simulink model "SMC2"  (R2018b)
settings: Solver=VariableStepAuto  StartTime=0.0  StopTime=50  MaxStep=0.001  RelTol=1e-3  EnableMultiTasking=on
settings Model: Creator=omid_zandi  LastModifiedBy=Arash
settings OptimizationCC: LifeSpan=inf
settings DebuggingCC: SFUnexpectedBacktrackingDiag=warning  SFNoUnconditionalDefaultTransitionDiag=warning
settings SFSimCC: SimUseLocalCustomCode=off
settings RTWCC: RTWUseLocalCustomCode=off
settings CodeAppCC: StateflowObjectComments=on
settings GRTTargetCC: TargetLangStandard=C89/C90 (ANSI)  GeneratePreprocessorConditionals=Disable all
settings ConfigComp: CovMetricSettings=dw  CovHtmlReporting=on  CovSaveCumulativeToWorkspaceVar=on  CovSaveSingleToWorkspaceVar=on  CovExternalEMLEnable=off

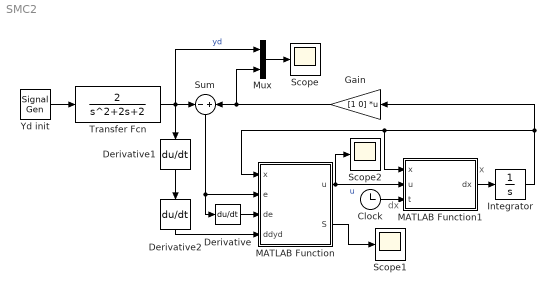
== system SMC2 ==
  note: dx
  note: x
  Clock : Clock
  Derivative : Derivative
  Derivative1 : Derivative
  Derivative2 : Derivative
  Gain : Gain  Gain=[1 0]  Multiplication=Matrix(K*u)
  Integrator : Integrator  InitialCondition=randn(2,1)
  MATLAB Function : MATLAB Function  TreatAsAtomicUnit=on
  MATLAB Function1 : MATLAB Function  TreatAsAtomicUnit=on
  Mux : Mux  Inputs=2
  Scope : Scope
  Scope1 : Scope
  Scope2 : Scope
  Sum : Sum  Inputs=-|+
  Transfer Fcn : TransferFcn  Numerator=[2]  Denominator="[1  2 2]"
  "Yd init " : SignalGenerator  WaveForm=square  Frequency=0.05
  wires:
  Integrator/1 -> MATLAB Function1/1(x), MATLAB Function/1(x), Gain/1
  MATLAB Function1/1(dx) -> Integrator/1
  MATLAB Function/1(u) -> Scope2/1, MATLAB Function1/2(u)  "u"
  Clock/1 -> MATLAB Function1/3(t)
  "Yd init "/1 -> Transfer Fcn/1
  Transfer Fcn/1 -> Mux/1, Derivative1/1, Sum/1  "yd"
  Gain/1 -> Mux/2, Sum/2
  Sum/1 -> MATLAB Function/2(e), Derivative/1
  Derivative/1 -> MATLAB Function/3(de)
  Derivative1/1 -> Derivative2/1
  Derivative2/1 -> MATLAB Function/4(ddyd)
  MATLAB Function/2(S) -> Scope1/1
  Mux/1 -> Scope/1

== matlab function SMC2/MATLAB Function1 ==
  data: x input; dx output; u input; t input
function dx = fcn(x , u , t)
%#codegen
dx = zeros(2,1) ;
dx(1) = x(2) ; 
dx(2) = x(1) * exp(-x(2)^2) + (1.5 + sin(t))*u ;

== matlab function SMC2/MATLAB Function ==
  data: x input; u output; S output; e input; de input; ddyd input
function [u , S] = fcn(x, e, de, ddyd)
k = 4;
eta = 4;
EPS = 0.01;
S = de  + k * e;
F = (abs(x(1)) + k * abs(x(2)) + abs(ddyd))/0.5;
% u = -(F + eta) * sign(S);
% u = -(F + eta) * S/(abs(S)  + EPS);
u = -(F + eta) * SAT(S);
end

% To avoid chattering
function  Z = SAT(S)
delta = 0.1;
if S > delta
    Z = 1;
elseif S < -delta
    Z = -1;
else
    Z = 1/delta * S;
end
end
